simulink model "gm_uz_pmsm_model_9ph_vnl"  (R2021b)
settings: Solver=FixedStepAuto  StartTime=0.0  StopTime=0.8  RelTol=1e-3
PreLoadFcn:
  | uz_pmsm_model_9ph_init_parameter
undefined symbols (not defined in the file or in its folder): a, b, c, friction_coefficient, inertia, k_i_d, k_i_q, k_p_d, k_p_q, Kpd, L_d, L_o1, L_o2, L_q, L_x1, L_x2, L_y1, L_y2, L_zero, polepair, psi_pm, R_1, static_friction_torque, Tnd, ts
libraries: hdlmdlgenlib x191, hdlsllib x90, dspsigops x19, simulink x17, slpidlib x2, spsAlphaBetaZerotodq0Lib x1, pid_lib x1, spsdq0toAlphaBetaZeroLib x1
(part 4 of 7)

== system gm_uz_pmsm_model_9ph_vnl/uz_pmsm_model_9ph/Line-Line to Phase voltage1 ==
  In1 : Inport  OutDataTypeStr=single  PortDimensions=[3]  SampleTime=1e-08
  Complex to Real-Imag : ComplexToRealImag  SampleTime=1e-08
  Constant : Constant  Value=single(0)  OutDataTypeStr=single  SampleTime=1e-08
  Constant1 : Constant  Value=complex(0.5, -0.28867512941360474)  OutDataTypeStr=single  SampleTime=1e-08
  Product : Subsystem
      mask Display: disp('NFP\nmul');
  Product1 : Subsystem
      mask Display: disp('NFP\nmul');
  Product2 : Subsystem
      mask Display: disp('NFP\nmul');
  Product3 : Subsystem
      mask Display: disp('NFP\nmul');
  Product_AC_minus_BD : Subsystem
      mask Display: disp('NFP\nadd');
  Product_AD_plus_BC : Subsystem
      mask Display: disp('NFP\nadd');
  Product_C2ReIm_1 : ComplexToRealImag  SampleTime=1e-08
  Product_C2ReIm_2 : ComplexToRealImag  SampleTime=1e-08
  Product_ReIm2Complex : RealImagToComplex  SampleTime=1e-08
  Real-Imag to Complex : RealImagToComplex  ConstantPart=single(0)  SampleTime=1e-08
  abc   to   alpha_beta_0 : Subsystem
  abc   to   alpha_beta_0_out1_2_term2 : Terminator
  alpha_beta_0   to   abc : Subsystem
  delayMatch{,1..3} (4 alike) : Delay  DelayLength=double(24)  InitialCondition=0  SampleTime=1e-08
  mux : Mux  Inputs=3
  t : Demux  Outputs=3
  Out1 : Outport  SampleTime=1e-08
  wires:
  In1/1 -> abc   to   alpha_beta_0/1("a, b, c")
  Product_AD_plus_BC/1(Out1) -> Product_ReIm2Complex/2
  Product_AC_minus_BD/1(Out1) -> Product_ReIm2Complex/1
  Product3/1(Out1) -> Product_AD_plus_BC/2(In2)
  Product2/1(Out1) -> Product_AC_minus_BD/2(In2)
  Product1/1(Out1) -> Product_AD_plus_BC/1(In1)
  Product/1(Out1) -> Product_AC_minus_BD/1(In1)
  Product_C2ReIm_2/1 -> delayMatch/1, delayMatch3/1
  Product_C2ReIm_2/2 -> delayMatch1/1, delayMatch2/1
  delayMatch2/1 -> Product2/2(In2)
  delayMatch3/1 -> Product3/2(In2)
  delayMatch1/1 -> Product1/2(In2)
  delayMatch/1 -> Product/2(In2)
  Product_C2ReIm_1/2 -> Product2/1(In1), Product3/1(In1)
  Product_C2ReIm_1/1 -> Product/1(In1), Product1/1(In1)
  t/3 -> abc   to   alpha_beta_0_out1_2_term2/1
  t/2 -> Real-Imag to Complex/2
  t/1 -> Real-Imag to Complex/1
  alpha_beta_0   to   abc/1("a, b, c") -> Out1/1
  abc   to   alpha_beta_0/1("alpha, beta, 0 ") -> t/1
  Real-Imag to Complex/1 -> Product_C2ReIm_1/1
  Product_ReIm2Complex/1 -> Complex to Real-Imag/1
  mux/1 -> alpha_beta_0   to   abc/1("alpha, beta, 0  ")
  Constant1/1 -> Product_C2ReIm_2/1
  Constant/1 -> mux/3
  Complex to Real-Imag/2 -> mux/2
  Complex to Real-Imag/1 -> mux/1

== system gm_uz_pmsm_model_9ph_vnl/uz_pmsm_model_9ph/Line-Line to Phase voltage2 ==
  In1 : Inport  OutDataTypeStr=single  PortDimensions=[3]  SampleTime=1e-08
  Complex to Real-Imag : ComplexToRealImag  SampleTime=1e-08
  Constant : Constant  Value=single(0)  OutDataTypeStr=single  SampleTime=1e-08
  Constant1 : Constant  Value=complex(0.5, -0.28867512941360474)  OutDataTypeStr=single  SampleTime=1e-08
  Product : Subsystem
      mask Display: disp('NFP\nmul');
  Product1 : Subsystem
      mask Display: disp('NFP\nmul');
  Product2 : Subsystem
      mask Display: disp('NFP\nmul');
  Product3 : Subsystem
      mask Display: disp('NFP\nmul');
  Product_AC_minus_BD : Subsystem
      mask Display: disp('NFP\nadd');
  Product_AD_plus_BC : Subsystem
      mask Display: disp('NFP\nadd');
  Product_C2ReIm_1 : ComplexToRealImag  SampleTime=1e-08
  Product_C2ReIm_2 : ComplexToRealImag  SampleTime=1e-08
  Product_ReIm2Complex : RealImagToComplex  SampleTime=1e-08
  Real-Imag to Complex : RealImagToComplex  ConstantPart=single(0)  SampleTime=1e-08
  abc   to   alpha_beta_0 : Subsystem
  abc   to   alpha_beta_0_out1_2_term2 : Terminator
  alpha_beta_0   to   abc : Subsystem
  delayMatch{,1..3} (4 alike) : Delay  DelayLength=double(24)  InitialCondition=0  SampleTime=1e-08
  mux : Mux  Inputs=3
  t : Demux  Outputs=3
  Out1 : Outport  SampleTime=1e-08
  wires:
  In1/1 -> abc   to   alpha_beta_0/1("a, b, c")
  Product_AD_plus_BC/1(Out1) -> Product_ReIm2Complex/2
  Product_AC_minus_BD/1(Out1) -> Product_ReIm2Complex/1
  Product3/1(Out1) -> Product_AD_plus_BC/2(In2)
  Product2/1(Out1) -> Product_AC_minus_BD/2(In2)
  Product1/1(Out1) -> Product_AD_plus_BC/1(In1)
  Product/1(Out1) -> Product_AC_minus_BD/1(In1)
  Product_C2ReIm_2/1 -> delayMatch/1, delayMatch3/1
  Product_C2ReIm_2/2 -> delayMatch1/1, delayMatch2/1
  delayMatch2/1 -> Product2/2(In2)
  delayMatch3/1 -> Product3/2(In2)
  delayMatch1/1 -> Product1/2(In2)
  delayMatch/1 -> Product/2(In2)
  Product_C2ReIm_1/2 -> Product2/1(In1), Product3/1(In1)
  Product_C2ReIm_1/1 -> Product/1(In1), Product1/1(In1)
  t/3 -> abc   to   alpha_beta_0_out1_2_term2/1
  t/2 -> Real-Imag to Complex/2
  t/1 -> Real-Imag to Complex/1
  alpha_beta_0   to   abc/1("a, b, c") -> Out1/1
  abc   to   alpha_beta_0/1("alpha, beta, 0 ") -> t/1
  Real-Imag to Complex/1 -> Product_C2ReIm_1/1
  Product_ReIm2Complex/1 -> Complex to Real-Imag/1
  mux/1 -> alpha_beta_0   to   abc/1("alpha, beta, 0  ")
  Constant1/1 -> Product_C2ReIm_2/1
  Constant/1 -> mux/3
  Complex to Real-Imag/2 -> mux/2
  Complex to Real-Imag/1 -> mux/1

== system gm_uz_pmsm_model_9ph_vnl/uz_pmsm_model_9ph/Product ==
  In1 : Inport
  In2 : Inport  Port=2
  Product : Product  Inputs=**  OutDataTypeStr=double  SampleTime=1e-08
  Product_pd1 : Delay  DelayLength=6
  Out1 : Outport
  wires:
  Product_pd1/1 -> Out1/1
  Product/1 -> Product_pd1/1
  In2/1 -> Product/2
  In1/1 -> Product/1

== system gm_uz_pmsm_model_9ph_vnl/uz_pmsm_model_9ph/Product1 ==
  In1 : Inport
  In2 : Inport  Port=2
  Product1 : Product  Inputs=**  OutDataTypeStr=double  SampleTime=1e-08
  Product1_pd1 : Delay  DelayLength=6
  Out1 : Outport
  wires:
  Product1_pd1/1 -> Out1/1
  Product1/1 -> Product1_pd1/1
  In2/1 -> Product1/2
  In1/1 -> Product1/1

== system gm_uz_pmsm_model_9ph_vnl/uz_pmsm_model_9ph/Product10 ==
  In1 : Inport
  In2 : Inport  Port=2
  Product10 : Product  Inputs=**  OutDataTypeStr=double  SampleTime=1e-08
  Product10_pd1 : Delay  DelayLength=6
  Out1 : Outport
  wires:
  Product10_pd1/1 -> Out1/1
  Product10/1 -> Product10_pd1/1
  In2/1 -> Product10/2
  In1/1 -> Product10/1

== system gm_uz_pmsm_model_9ph_vnl/uz_pmsm_model_9ph/Product11 ==
  In1 : Inport
  In2 : Inport  Port=2
  Product11 : Product  Inputs=**  OutDataTypeStr=single  SampleTime=1e-08
  Product11_pd1 : Delay  DelayLength=6
  Out1 : Outport
  wires:
  Product11_pd1/1 -> Out1/1
  Product11/1 -> Product11_pd1/1
  In2/1 -> Product11/2
  In1/1 -> Product11/1

== system gm_uz_pmsm_model_9ph_vnl/uz_pmsm_model_9ph/Product2 ==
  In1 : Inport
  In2 : Inport  Port=2
  Product2 : Product  Inputs=**  OutDataTypeStr=single  SampleTime=1e-08
  Product2_pd1 : Delay  DelayLength=6
  Out1 : Outport
  wires:
  Product2_pd1/1 -> Out1/1
  Product2/1 -> Product2_pd1/1
  In2/1 -> Product2/2
  In1/1 -> Product2/1

== system gm_uz_pmsm_model_9ph_vnl/uz_pmsm_model_9ph/Product3 ==
  In1 : Inport
  In2 : Inport  Port=2
  Product3 : Product  Inputs=**  OutDataTypeStr=single  SampleTime=1e-08
  Product3_pd1 : Delay  DelayLength=6
  Out1 : Outport
  wires:
  Product3_pd1/1 -> Out1/1
  Product3/1 -> Product3_pd1/1
  In2/1 -> Product3/2
  In1/1 -> Product3/1

== system gm_uz_pmsm_model_9ph_vnl/uz_pmsm_model_9ph/Product5 ==
  In1 : Inport
  In2 : Inport  Port=2
  Product5 : Product  Inputs=**  OutDataTypeStr=double  SampleTime=1e-08
  Product5_pd1 : Delay  DelayLength=6
  Out1 : Outport
  wires:
  Product5_pd1/1 -> Out1/1
  Product5/1 -> Product5_pd1/1
  In2/1 -> Product5/2
  In1/1 -> Product5/1

== system gm_uz_pmsm_model_9ph_vnl/uz_pmsm_model_9ph/Product6 ==
  In1 : Inport
  In2 : Inport  Port=2
  Product6 : Product  Inputs=**  OutDataTypeStr=double  SampleTime=1e-08
  Product6_pd1 : Delay  DelayLength=6
  Out1 : Outport
  wires:
  Product6_pd1/1 -> Out1/1
  Product6/1 -> Product6_pd1/1
  In2/1 -> Product6/2
  In1/1 -> Product6/1

== system gm_uz_pmsm_model_9ph_vnl/uz_pmsm_model_9ph/Product7 ==
  In1 : Inport
  In2 : Inport  Port=2
  Product7 : Product  Inputs=**  OutDataTypeStr=double  SampleTime=1e-08
  Product7_pd1 : Delay  DelayLength=6
  Out1 : Outport
  wires:
  Product7_pd1/1 -> Out1/1
  Product7/1 -> Product7_pd1/1
  In2/1 -> Product7/2
  In1/1 -> Product7/1

== system gm_uz_pmsm_model_9ph_vnl/uz_pmsm_model_9ph/Product8 ==
  In1 : Inport
  In2 : Inport  Port=2
  Product8 : Product  Inputs=**  OutDataTypeStr=double  SampleTime=1e-08
  Product8_pd1 : Delay  DelayLength=6
  Out1 : Outport
  wires:
  Product8_pd1/1 -> Out1/1
  Product8/1 -> Product8_pd1/1
  In2/1 -> Product8/2
  In1/1 -> Product8/1

== system gm_uz_pmsm_model_9ph_vnl/uz_pmsm_model_9ph/Product9 ==
  In1 : Inport
  In2 : Inport  Port=2
  Product9 : Product  Inputs=**  OutDataTypeStr=single  SampleTime=1e-08
  Product9_pd1 : Delay  DelayLength=6
  Out1 : Outport
  wires:
  Product9_pd1/1 -> Out1/1
  Product9/1 -> Product9_pd1/1
  In2/1 -> Product9/2
  In1/1 -> Product9/1

== system gm_uz_pmsm_model_9ph_vnl/uz_pmsm_model_9ph/Sine_Cosine ==
  In1 : Inport
  Sine_Cosine : Trigonometry  Operator=sincos  SampleTime=1e-08
  Sine_Cosine_pd1 : Delay  DelayLength=27
  Sine_Cosine_pd2 : Delay  DelayLength=27
  Out1 : Outport
  Out2 : Outport  Port=2
  wires:
  Sine_Cosine_pd2/1 -> Out2/1
  Sine_Cosine/2 -> Sine_Cosine_pd2/1
  Sine_Cosine_pd1/1 -> Out1/1
  Sine_Cosine/1 -> Sine_Cosine_pd1/1
  In1/1 -> Sine_Cosine/1

== system gm_uz_pmsm_model_9ph_vnl/uz_pmsm_model_9ph/Sum1 ==
  In1 : Inport
  In2 : Inport  Port=2
  Sum1 : Sum  OutDataTypeStr=single  SampleTime=1e-08
  Sum1_pd1 : Delay  DelayLength=6
  Out1 : Outport
  wires:
  Sum1_pd1/1 -> Out1/1
  Sum1/1 -> Sum1_pd1/1
  In2/1 -> Sum1/2
  In1/1 -> Sum1/1

== system gm_uz_pmsm_model_9ph_vnl/uz_pmsm_model_9ph/Sum1_stage2 ==
  In1 : Inport
  In2 : Inport  Port=2
  Sum1_stage2 : Sum  Inputs=+-  OutDataTypeStr=double  SampleTime=1e-08
  Sum1_stage2_pd1 : Delay  DelayLength=6
  Out1 : Outport
  wires:
  Sum1_stage2_pd1/1 -> Out1/1
  Sum1_stage2/1 -> Sum1_stage2_pd1/1
  In2/1 -> Sum1_stage2/2
  In1/1 -> Sum1_stage2/1

== system gm_uz_pmsm_model_9ph_vnl/uz_pmsm_model_9ph/Sum1_stage3 ==
  In1 : Inport
  In2 : Inport  Port=2
  Sum1_stage3 : Sum  Inputs=+-  OutDataTypeStr=double  SampleTime=1e-08
  Sum1_stage3_pd1 : Delay  DelayLength=6
  Out1 : Outport
  wires:
  Sum1_stage3_pd1/1 -> Out1/1
  Sum1_stage3/1 -> Sum1_stage3_pd1/1
  In2/1 -> Sum1_stage3/2
  In1/1 -> Sum1_stage3/1

== system gm_uz_pmsm_model_9ph_vnl/uz_pmsm_model_9ph/Sum2 ==
  In1 : Inport
  In2 : Inport  Port=2
  Sum2 : Sum  Inputs=+-  OutDataTypeStr=double  SampleTime=1e-08
  Sum2_pd1 : Delay  DelayLength=6
  Out1 : Outport
  wires:
  Sum2_pd1/1 -> Out1/1
  Sum2/1 -> Sum2_pd1/1
  In2/1 -> Sum2/2
  In1/1 -> Sum2/1

== system gm_uz_pmsm_model_9ph_vnl/uz_pmsm_model_9ph/Sum3 ==
  In1 : Inport
  In2 : Inport  Port=2
  Sum3 : Sum  OutDataTypeStr=double  SampleTime=1e-08
  Sum3_pd1 : Delay  DelayLength=6
  Out1 : Outport
  wires:
  Sum3_pd1/1 -> Out1/1
  Sum3/1 -> Sum3_pd1/1
  In2/1 -> Sum3/2
  In1/1 -> Sum3/1

== system gm_uz_pmsm_model_9ph_vnl/uz_pmsm_model_9ph/Sum31 ==
  In1 : Inport
  In2 : Inport  Port=2
  Sum31 : Sum  OutDataTypeStr=double  SampleTime=1e-08
  Sum31_pd1 : Delay  DelayLength=6
  Out1 : Outport
  wires:
  Sum31_pd1/1 -> Out1/1
  Sum31/1 -> Sum31_pd1/1
  In2/1 -> Sum31/2
  In1/1 -> Sum31/1

== system gm_uz_pmsm_model_9ph_vnl/uz_pmsm_model_9ph/Sum310 ==
  In1 : Inport
  In2 : Inport  Port=2
  Sum310 : Sum  OutDataTypeStr=double  SampleTime=1e-08
  Sum310_pd1 : Delay  DelayLength=6
  Out1 : Outport
  wires:
  Sum310_pd1/1 -> Out1/1
  Sum310/1 -> Sum310_pd1/1
  In2/1 -> Sum310/2
  In1/1 -> Sum310/1

== system gm_uz_pmsm_model_9ph_vnl/uz_pmsm_model_9ph/Sum32 ==
  In1 : Inport
  In2 : Inport  Port=2
  Sum32 : Sum  OutDataTypeStr=double  SampleTime=1e-08
  Sum32_pd1 : Delay  DelayLength=6
  Out1 : Outport
  wires:
  Sum32_pd1/1 -> Out1/1
  Sum32/1 -> Sum32_pd1/1
  In2/1 -> Sum32/2
  In1/1 -> Sum32/1

== system gm_uz_pmsm_model_9ph_vnl/uz_pmsm_model_9ph/Sum33 ==
  In1 : Inport
  In2 : Inport  Port=2
  Sum33 : Sum  Inputs=+-  OutDataTypeStr=single  SampleTime=1e-08
  Sum33_pd1 : Delay  DelayLength=6
  Out1 : Outport
  wires:
  Sum33_pd1/1 -> Out1/1
  Sum33/1 -> Sum33_pd1/1
  In2/1 -> Sum33/2
  In1/1 -> Sum33/1

== system gm_uz_pmsm_model_9ph_vnl/uz_pmsm_model_9ph/Sum34 ==
  In1 : Inport
  In2 : Inport  Port=2
  Sum34 : Sum  OutDataTypeStr=double  SampleTime=1e-08
  Sum34_pd1 : Delay  DelayLength=6
  Out1 : Outport
  wires:
  Sum34_pd1/1 -> Out1/1
  Sum34/1 -> Sum34_pd1/1
  In2/1 -> Sum34/2
  In1/1 -> Sum34/1

== system gm_uz_pmsm_model_9ph_vnl/uz_pmsm_model_9ph/Sum35 ==
  In1 : Inport
  In2 : Inport  Port=2
  Sum35 : Sum  OutDataTypeStr=double  SampleTime=1e-08
  Sum35_pd1 : Delay  DelayLength=6
  Out1 : Outport
  wires:
  Sum35_pd1/1 -> Out1/1
  Sum35/1 -> Sum35_pd1/1
  In2/1 -> Sum35/2
  In1/1 -> Sum35/1

== system gm_uz_pmsm_model_9ph_vnl/uz_pmsm_model_9ph/Sum36 ==
  In1 : Inport
  In2 : Inport  Port=2
  Sum36 : Sum  OutDataTypeStr=double  SampleTime=1e-08
  Sum36_pd1 : Delay  DelayLength=6
  Out1 : Outport
  wires:
  Sum36_pd1/1 -> Out1/1
  Sum36/1 -> Sum36_pd1/1
  In2/1 -> Sum36/2
  In1/1 -> Sum36/1

== system gm_uz_pmsm_model_9ph_vnl/uz_pmsm_model_9ph/Sum37 ==
  In1 : Inport
  In2 : Inport  Port=2
  Sum37 : Sum  OutDataTypeStr=double  SampleTime=1e-08
  Sum37_pd1 : Delay  DelayLength=6
  Out1 : Outport
  wires:
  Sum37_pd1/1 -> Out1/1
  Sum37/1 -> Sum37_pd1/1
  In2/1 -> Sum37/2
  In1/1 -> Sum37/1

== system gm_uz_pmsm_model_9ph_vnl/uz_pmsm_model_9ph/Sum38 ==
  In1 : Inport
  In2 : Inport  Port=2
  Sum38 : Sum  OutDataTypeStr=double  SampleTime=1e-08
  Sum38_pd1 : Delay  DelayLength=6
  Out1 : Outport
  wires:
  Sum38_pd1/1 -> Out1/1
  Sum38/1 -> Sum38_pd1/1
  In2/1 -> Sum38/2
  In1/1 -> Sum38/1

== system gm_uz_pmsm_model_9ph_vnl/uz_pmsm_model_9ph/Sum39 ==
  In1 : Inport
  In2 : Inport  Port=2
  Sum39 : Sum  OutDataTypeStr=double  SampleTime=1e-08
  Sum39_pd1 : Delay  DelayLength=6
  Out1 : Outport
  wires:
  Sum39_pd1/1 -> Out1/1
  Sum39/1 -> Sum39_pd1/1
  In2/1 -> Sum39/2
  In1/1 -> Sum39/1

== system gm_uz_pmsm_model_9ph_vnl/uz_pmsm_model_9ph/Sum_stage2 ==
  In1 : Inport
  In2 : Inport  Port=2
  Sum_stage2 : Sum  Inputs=+-  OutDataTypeStr=double  SampleTime=1e-08
  Sum_stage2_pd1 : Delay  DelayLength=6
  Out1 : Outport
  wires:
  Sum_stage2_pd1/1 -> Out1/1
  Sum_stage2/1 -> Sum_stage2_pd1/1
  In2/1 -> Sum_stage2/2
  In1/1 -> Sum_stage2/1

== system gm_uz_pmsm_model_9ph_vnl/uz_pmsm_model_9ph/Sum_stage3 ==
  In1 : Inport
  In2 : Inport  Port=2
  Sum_stage3 : Sum  OutDataTypeStr=double  SampleTime=1e-08
  Sum_stage3_pd1 : Delay  DelayLength=6
  Out1 : Outport
  wires:
  Sum_stage3_pd1/1 -> Out1/1
  Sum_stage3/1 -> Sum_stage3_pd1/1
  In2/1 -> Sum_stage3/2
  In1/1 -> Sum_stage3/1
